simulink model "model"  (R2024a)
settings: Solver=FixedStepAuto  StartTime=0.0  StopTime=10.0  FixedStep=0.001  RelTol=1e-3
settings Model: Creator=Professional  LastModifiedBy=Professional

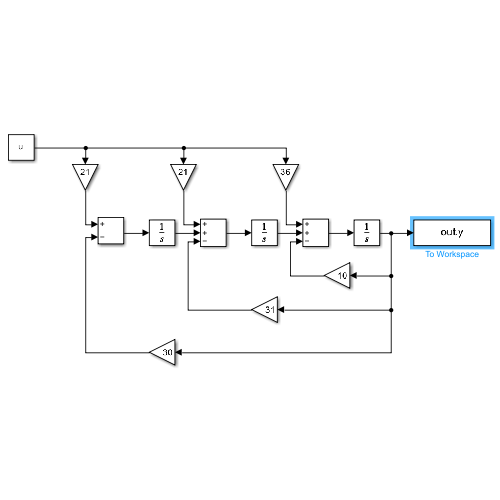
[thumbnail: Simulink's stored preview of the top-level diagram]
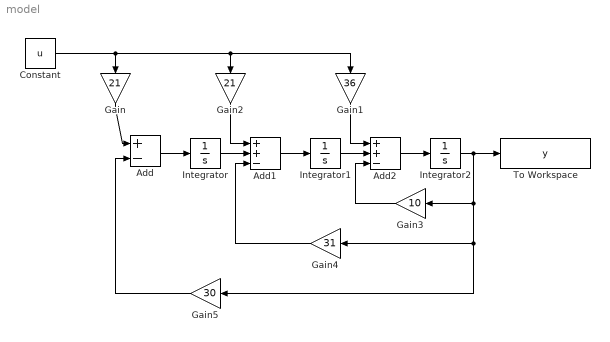
== system model ==
  Add : Sum  Inputs=+-
  Add1 : Sum  Inputs=++-
  Add2 : Sum  Inputs=++-
  Constant : Constant  Value=u
  Gain : Gain  Gain=21
  Gain1 : Gain  Gain=36
  Gain2 : Gain  Gain=21
  Gain3 : Gain  Gain=10
  Gain4 : Gain  Gain=31
  Gain5 : Gain  Gain=30
  Integrator : Integrator
  Integrator1 : Integrator
  Integrator2 : Integrator
  To Workspace : ToWorkspace  VariableName=y  SaveFormat=Timeseries  SampleTime=-1
  wires:
  Constant/1 -> Gain1/1, Gain2/1, Gain/1
  Gain/1 -> Add/1
  Add/1 -> Integrator/1
  Integrator/1 -> Add1/2
  Gain2/1 -> Add1/1
  Add1/1 -> Integrator1/1
  Gain1/1 -> Add2/1
  Integrator1/1 -> Add2/2
  Add2/1 -> Integrator2/1
  Gain3/1 -> Add2/3
  Gain4/1 -> Add1/3
  Gain5/1 -> Add/2
  Integrator2/1 -> To Workspace/1, Gain3/1, Gain4/1, Gain5/1
